simulink model "q_four_awmat"  (R2019b)
settings: Solver=VariableStepAuto  StartTime=0.0  StopTime=5  RelTol=1e-3
values from neighbouring files (symbols this model uses):
  A_fs = [-0.5 0 -455;0 -2.9 455; 1 -1 0]    [ex4.m]    (also in ex5.m; ex5test.m)
  B_fs = [17 0; 0 -5; 0 0]    [ex4.m]    (also in ex5.m; ex5test.m)
  C_fs = [1 0 0; 0 1 0; 0 0 1]    [ex4.m]    (also in ex5.m; ex5test.m)
  D_fs = [0 0;0 0; 0 0]    [ex4.m]    (also in ex5.m; ex5test.m)
  kq4 = place(A4, B4, p4)    [ex4.m]    (also in ex5.m; ex5test.m)
settings Model: Creator=rafek  LastModifiedBy=rafek

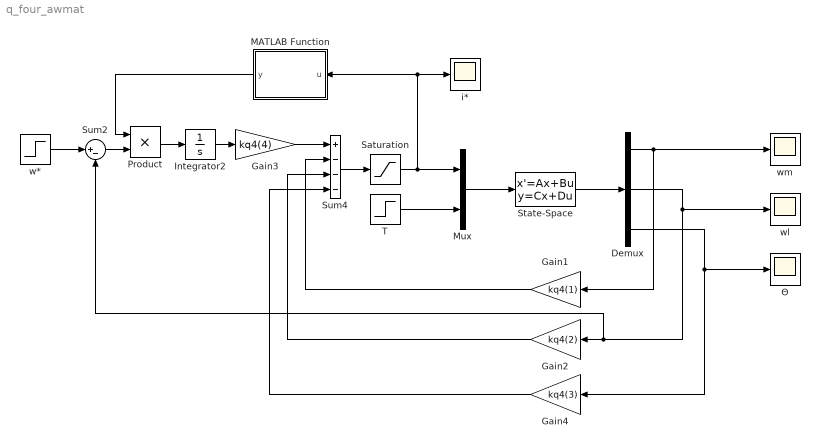
== system q_four_awmat ==
  Demux : Demux  Outputs=3
  Gain1 : Gain  Gain=kq4(1)
  Gain2 : Gain  Gain=kq4(2)
  Gain3 : Gain  Gain=kq4(4)
  Gain4 : Gain  Gain=kq4(3)
  Integrator2 : Integrator
  MATLAB Function : MATLAB Function  TreatAsAtomicUnit=on
  Mux : Mux  Inputs=2
  Product : Product
  Saturation : Saturate  UpperLimit=42  LowerLimit=-42
  State-Space : StateSpace  A=A_fs  B=B_fs  C=C_fs  D=D_fs  InitialCondition=0
  Sum2 : Sum  Inputs=|+-
  Sum4 : Sum  Inputs=+---
  T : Step  Time=0  After=75  SampleTime=0
  i* : Scope
  w* : Step  Time=0  After=100  SampleTime=0
  wl : Scope
  wm : Scope
  Θ : Scope
  wires:
  w*/1 -> Sum2/1
  Gain1/1 -> Sum4/2
  T/1 -> Mux/2
  Gain3/1 -> Sum4/1
  Sum2/1 -> Product/2
  Mux/1 -> State-Space/1
  Product/1 -> Integrator2/1
  State-Space/1 -> Demux/1
  MATLAB Function/1(y) -> Product/1
  Gain2/1 -> Sum4/3
  Gain4/1 -> Sum4/4
  Demux/2 -> Sum2/2, Gain2/1, wl/1
  Demux/1 -> Gain1/1, wm/1
  Integrator2/1 -> Gain3/1
  Demux/3 -> Gain4/1, Θ/1
  Sum4/1 -> Saturation/1
  Saturation/1 -> i*/1, MATLAB Function/1(u), Mux/1

== matlab function q_four_awmat/MATLAB Function ==
  data: u input; y output
function y = fcn(u)
if u>42 || u<0
    y=0;
else
    y=1;
end
end
